simulink model "modelo_planta_CODESYS"  (R2025b)
settings: Solver=FixedStepAuto  StartTime=0.0  StopTime=inf  FixedStep=Ts2  MaxStep=1e-3  RelTol=1e-3
undefined symbols (not defined in the file): ah_max, at_max, bcx, bcy, bh_eq, bhb, bhEb, bhwu, bt, bt_eq, btb, btw, g, Hc, ih, it, Jh_eq, Jt_eq, Kcy, khwu, Ki_h, Ki_t, Kp_h, Kp_t, Kpos_h, Kpos_t, Ktw, lambda, Lh, Lh0, lh_0, Lt, magnitude, Mc_max, Ms, Mt, rhd, rtd, tau_hm, tau_tm, Thb_Max, ThEb_Max, Thm_0, Thm_Max, titahm_0, titatm_0, Ts0, Ts1, Ts2, Ttb_Max, Ttm_0, Ttm_Max, vh_0, vlx_0, vly_0, vt_0, vt_max, Wc, whm_0, whm_rated ... (+11)
libraries: simulink x10, opcualib x7, sl3dlib x1, simulink_extras x1, dspnetwork x1
(part 1 of 2)
settings Model: SimulationMode=accelerator  Creator=Nahuel  LastModifiedBy=nahue
settings SolverCC: ZeroCrossControl=DisableAll
settings DebuggingCC: UnderSpecifiedDimensionMsg=warning
settings SFSimCC: SimTargetLang=C++  SimDLTargetLibrary=mkl-dnn
settings RTWCC: GPUComputeCapability=3.5

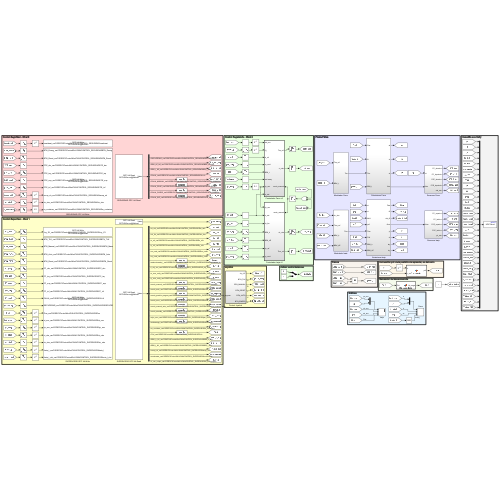
[thumbnail: Simulink's stored preview of the top-level diagram]
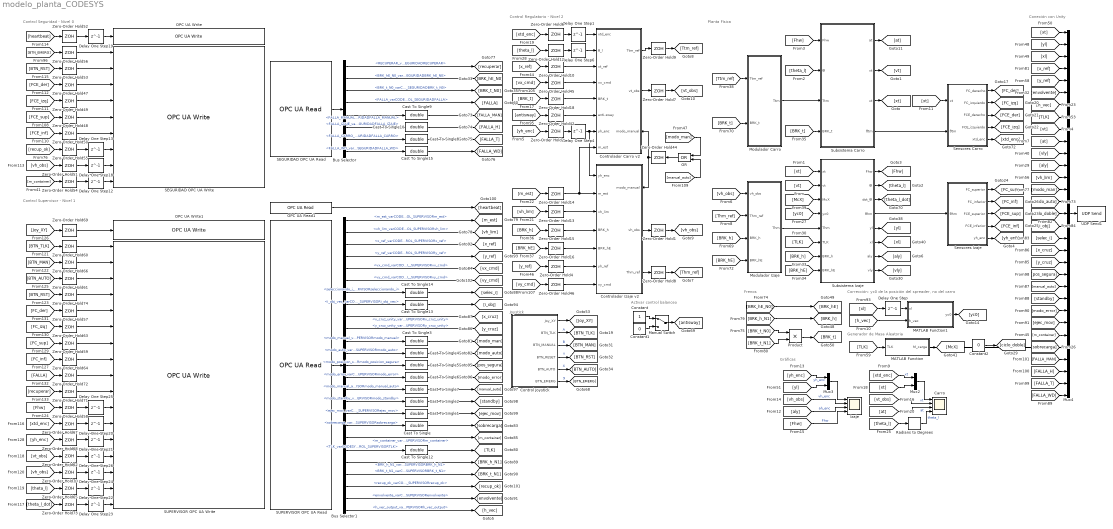
== system modelo_planta_CODESYS ==
  note: Activar control balanceo
  note: Generador de Masa Aleatoria
  note: Frenos
  note: Corrección: yc0 de la posición del spreader, no del carro
  note: Joystick
  note: Control Regulatorio - Nivel 2
  note: Conexión con Unity
  note: Planta Física
  note: Gráficas
  note: Control Seguridad - Nivel 0
  note: Control Supervisor - Nivel 1
  Bus Selector : BusSelector  OutputSignals=RECUPERAR_varCODESYSControlWinV3X64CONTROL_SEGURIDADRECUPERAR,BRK_hE_N0_varCODESYSControlWinV3X64CONTROL_SEGURIDADBRK_hE_N0,BRK_t_N0_varCODESYSControlWinV3X64CONTROL_SEGURIDADBRK_t_N0,FALLA_varCODESYSControlWinV3X64CONTROL_SEGURIDADFALLA,FALLA_MANUAL_varCODESYSControlWinV3X64CONTROL_SEGURIDADFALLA_MANUAL,FALLA_IZAJE_varCODESYSControlWinV3X64CONTROL_SEGURIDADFALLA_IZAJE,FALLA_CARRO_varCODESYSControlWinV3X64CONTROL_SEGURIDADFALLA_CARRO,FALLA_WD_varCODESYSControlWinV3X64CONTROL_SEGURIDADFALLA_WD
  Bus Selector1 : BusSelector  OutputSignals=m_est_varCODESYSControlWinV3X64CONTROL_SUPERVISORm_est,vh_lim_varCODESYSControlWinV3X64CONTROL_SUPERVISORvh_lim,x_ref_varCODESYSControlWinV3X64CONTROL_SUPERVISORx_ref,y_ref_varCODESYSControlWinV3X64CONTROL_SUPERVISORy_ref,vx_cmd_varCODESYSControlWinV3X64CONTROL_SUPERVISORvx_cmd,vy_cmd_varCODESYSControlWinV3X64CONTROL_SUPERVISORvy_cmd,seleccionando_i_varCODESYSControlWinV3X64CONTROL_SUPERVISORseleccionando_i,i_obj_vec_varCODESYSControlWinV3X64CONTROL_SUPERVISORi_obj_vec,x_cruz_unity_varCODESYSControlWinV3X64CONTROL_SUPERVISORx_cruz_unity,y_cruz_unity_varCODESYSControlWinV3X64CONTROL_SUPERVISORy_cruz_unity,modo_manual_varCODESYSControlWinV3X64CONTROL_SUPERVISORmodo_manual,modo_auto_varCODESYSControlWinV3X64CONTROL_SUPERVISORmodo_auto,modo_posicion_segura_varCODESYSControlWinV3X64CONTROL_SUPERVISORmodo_posicion_segura,modo_error_varCODESYSControlWinV3X64CONTROL_SUPERVISORmodo_error,modo_manual_auto_varCODESYSControlWinV3X64CONTROL_SUPERVISORmodo_manual_auto,modo_standby_varCODESYSControlWinV3X64CONTROL_SUPERVISORmodo_standby,ejec_mov_varCODESYSControlWinV3X64CONTROL_SUPERVISORejec_mov,sobrecarga_varCODESYSControlWinV3X64CONTROL_SUPERVISORsobrecarga,m_container_varCODESYSControlWinV3X64CONTROL_SUPERVISORm_container,TLK_varCODESYSControlWinV3X64CONTROL_SUPERVISORTLK,BRK_h_N1_varCODESYSControlWinV3X64CONTROL_SUPERVISORBRK_h_N1,BRK_t_N1_varCODESYSControlWinV3X64CONTROL_SUPERVISORBRK_t_N1,recup_ok_varCODESYSControlWinV3X64CONTROL_SUPERVISORrecup_ok,envolvente_varCODESYSControlWinV3X64CONTROL_SUPERVISORenvolvente,h_vec_output_varCODESYSControlWinV3X64CONTROL_SUPERVISORh_vec_output
  Carro : Scope  NumInputPorts=4
      settings: AxesScalingNumUpdates=5  ActiveDisplayYMinimum=-26.90845  ActiveDisplayYMaximum=42.17601
  Cast To Single{,1..10,12..15} (15 alike) : DataTypeConversion  OutDataTypeStr=double  SaturateOnIntegerOverflow=off  RndMeth=Floor
  Constant : Constant
  Constant1 : Constant  Value=0
  Constant2 : Constant  Value=0
  "Control Joystick " : Subsystem  TreatAsAtomicUnit=on  SystemSampleTime=Ts2
  Controlador Carro v2 : Subsystem  Priority=3  TreatAsAtomicUnit=on  SystemSampleTime=Ts2
      settings: PortSchema="{\"entries\":[{\"content\":{\"sides\":[{\"content\":{\"connectorIds\":[\"In1\",\"In2\",\"In3\",\"In4\",\"In5\",\"In6\",\"In7\",\"In8\"]},\"type\":\"ConnectorPlacement.EquallySpacedRectSide\",\"uuid\":\"cec1db83-79e7-401c-9c5a-62bfe309052c\"},{\"content\":{\"connectorIds\":[\"Out1\",\"Out2\",\"In9\"],\"side\":\"RIGHT\"},\"type\":\"ConnectorPlacement.EquallySpacedRectSide\",\"uuid\":\"570b393c-e744-4def-bec0-7a29fbc05550\"},{\"content\":{\"side\":\"TOP\"},\"type\":\"ConnectorPlacement.EquallySpacedRectSide\",\"uuid\":\"ce77deb8-7996-49cb-8f1a-144112ebd13f\"}]},\"type\":\"ConnectorPlacement.EquallySpacedConnector\",\"uuid\":\"f3fbcf0d-9250-48f2-9b40-44fd72963ab4\"}],\"packageUris\":[\"http://schema.mathworks.com/mf0/Connector/R2020b\"],\"version\":\"1.0\"}"
  Controlador Izaje v2 : Subsystem  Priority=3  TreatAsAtomicUnit=on  SystemSampleTime=Ts2
      settings: PortSchema="{\"entries\":[{\"content\":{\"sides\":[{\"content\":{\"connectorIds\":[\"In1\",\"In2\",\"In3\",\"In4\",\"In5\",\"In6\",\"In7\"]},\"type\":\"ConnectorPlacement.EquallySpacedRectSide\",\"uuid\":\"22fc4638-29ab-445f-b4f3-d8ad1dc2dec6\"},{\"content\":{\"connectorIds\":[\"In8\",\"Out1\",\"Out2\"],\"side\":\"RIGHT\"},\"type\":\"ConnectorPlacement.EquallySpacedRectSide\",\"uuid\":\"5bc2e66a-532f-4a2d-8b33-72ae52e90077\"},{\"content\":{\"side\":\"TOP\"},\"type\":\"ConnectorPlacement.EquallySpacedRectSide\",\"uuid\":\"2db62695-ea1c-4a55-b954-e8d85fe38ca0\"}]},\"type\":\"ConnectorPlacement.EquallySpacedConnector\",\"uuid\":\"0df15d49-0909-4287-a965-a213712e4789\"}],\"packageUris\":[\"http://schema.mathworks.com/mf0/Connector/R2020b\"],\"version\":\"1.0\"}"
  Delay One Step : Delay  DelayLength=1  InitialCondition=xl_0
  Delay One Step1 : Delay  DelayLength=1  InitialCondition=xtd_0
  Delay One Step{6,12..13,18..19,22..24,26} (9 alike) : Delay  DelayLength=1  InitialCondition=0
  Delay One Step20 : Delay  DelayLength=1  InitialCondition=xt_0
  Delay One Step21 : Delay  DelayLength=1  InitialCondition=yh_0
  Delay One Step25 : Delay  DelayLength=1
  Delay One Step4 : Delay  DelayLength=1  InitialCondition=yh_0
  Izaje : Scope  NumInputPorts=4
      settings: ActiveDisplayYMinimum=-22.31965  ActiveDisplayYMaximum=45.47272
  MATLAB Function : MATLAB Function  TreatAsAtomicUnit=on
  MATLAB Function1 : MATLAB Function  TreatAsAtomicUnit=on
  Manual Switch : ManualSwitch
  Modulador Carro : Subsystem
  Modulador Izaje : Subsystem
  Mux2 : Mux  Inputs=2
  Mux3 : Mux  Inputs=2
  Mux4 : Mux  Inputs=31
  OPC UA Read1 : opcualib/OPC UA Read  SelectedServer=OPCUAServer@Nahuel  ServerList=OPCUAServer@Nahuel  NodeList={ '1', 'heartbeat', '4', '|var|CODESYS Control Win V3 x64.CONTROL_SUPERVISOR.heartbeat', '0' }  ShowQualityPort=off  ShowTimestampPort=off  ShowTimestampPortAs=Seconds since start  SampleTime=Ts1
  OPC UA Write : opcualib/OPC UA Write  SelectedServer=OPCUAServer@Nahuel  ServerList=OPCUAServer@Nahuel  SampleTime=Ts0  NodeList={ '1', 'heartbeat', '4', '|var|CODESYS Control Win V3 x64.CONTROL_SEGURIDAD.heartbeat', '0' }
  OPC UA Write1 : opcualib/OPC UA Write  SelectedServer=OPCUAServer@Nahuel  ServerList=OPCUAServer@Nahuel  SampleTime=Ts1  NodeList={ '1', 'Joy_XY', '4', '|var|CODESYS Control Win V3 x64.CONTROL_SUPERVISOR.Joy_XY', '0' }
  OR : Logic  Operator=OR  IconShape=distinctive  AllPortsSameDT=off  OutDataTypeStr=boolean
  Product : Product
  Radians to Degrees : simulink_extras/Transformations/Radians to Degrees
  SEGURIDAD OPC UA Read : opcualib/OPC UA Read  SelectedServer=OPCUAServer@Nahuel  ServerList=OPCUAServer@Nahuel  NodeList={ '1', 'RECUPERAR', '4', '|var|CODESYS Control Win V3 x64.CONTROL_SEGURIDAD.RECUPERAR', '0'; '2', 'BRK_hE_N0', '4', '|var|CODESYS Control Win V3 x64.CONTROL_SEGURIDAD.BRK_hE_N0', '0'; '3', 'BRK_t_N0', '4', '|var|CODESYS Control Win V3 x64.CONTROL_SEGURIDAD.BRK_t_N0', '0'; '4', 'FALLA', '4', '|var|CODESYS Control Win V3 x64.CONTROL_SEGURIDAD.FALLA', '0'; '5', 'FALLA_MANUAL', '4', '|var|CODESYS Control Win V3 x64.CONTROL_SEGURIDAD.FALLA_MANUAL', '0'; '6', 'FALLA_IZAJE', '4', '|var|CODESYS Control Win V3 x64.CONTROL_SEGURIDAD.FALLA_IZAJE', '0'; '7', 'FALLA_CARRO', '4', '|var|CODESYS Control Win V3 x64.CONTROL_SEGURIDAD.FALLA_CARRO', '0'; '8', 'FALLA_WD', '4', '|var|CODESYS Control Win V3 x64.CONTROL_SEGURIDAD.FALLA_WD', '0' }  ShowQualityPort=off  ShowTimestampPort=off  ShowTimestampPortAs=Seconds since start  SampleTime=0.1
  SEGURIDAD OPC UA Write : opcualib/OPC UA Write  SelectedServer=OPCUAServer@Nahuel  ServerList=OPCUAServer@Nahuel  SampleTime=0.1  NodeList={ '1', 'BTN_Emerg', '4', '|var|CODESYS Control Win V3 x64.CONTROL_SEGURIDAD.BTN_Emerg', '0'; '2', 'BTN_Reset', '4', '|var|CODESYS Control Win V3 x64.CONTROL_SEGURIDAD.BTN_Reset', '0'; '3', 'FCE_der', '4', '|var|CODESYS Control Win V3 x64.CONTROL_SEGURIDAD.FCE_der', '0'; '4', 'FCE_izq', '4', '|var|CODESYS Control Win V3 x64.CONTROL_SEGURIDAD.FCE_izq', '0'; '5', 'FCE_sup', '4', '|var|CODESYS Control Win V3 x64.CONTROL_SEGURIDAD.FCE_sup', '0'; '6', 'FCE_inf', '4', '|var|CODESYS Control Win V3 x64.CONTROL_SEGURIDAD.FCE_inf', '0'; '7', 'recup_ok', '4', '|var|CODESYS Control Win V3 x64.CONTROL_SEGURIDAD.recup_ok', '0'; '8', 'vh_obs', '4', '|var|CODESYS Control Win V3 x64.CONTROL_SEGURIDAD.vh_obs', '0'; '9', 'm_container', '4', '|var|CODESYS Control Win V3 x64.CONTROL_SEGURIDAD.m_container', '0' }
  SUPERVISOR OPC UA Read : opcualib/OPC UA Read  SelectedServer=OPCUAServer@Nahuel  ServerList=OPCUAServer@Nahuel  NodeList={ '1', 'm_est', '4', '|var|CODESYS Control Win V3 x64.CONTROL_SUPERVISOR.m_est', '0'; '2', 'vh_lim', '4', '|var|CODESYS Control Win V3 x64.CONTROL_SUPERVISOR.vh_lim', '0'; '3', 'x_ref', '4', '|var|CODESYS Control Win V3 x64.CONTROL_SUPERVISOR.x_ref', '0'; '4', 'y_ref', '4', '|var|CODESYS Control Win V3 x64.CONTROL_SUPERVISOR.y_ref', '0'; '5', 'vx_cmd', '4', '|var|CODESYS Control Win V3 x64.CONTROL_SUPERVISOR.vx_cmd', '0'; '6', 'vy_cmd', '4', '|var|CODESYS Control Win V3 x64.CONTROL_SUPERVISOR.vy_cmd', '0'; '7', 'seleccionando_i', '4', '|var|CODESYS Control Win V3 x64.CONTROL_SUPERVISOR.seleccionando_i', '0'; '8', 'i_obj_vec', '4', '|var|CODESYS Control Win V3 x64.CONTROL_SUPERVISOR.i_obj_vec', '0'; '9', 'x_cruz_unity', '4', '|var|CODESYS Control Win V3 x64.CONTROL_SUPERVISOR.x_cruz_unity', '0'; '10', 'y_cruz_unity', '4', '|var|CODESYS Control Win V3 x64.CONTROL_SUPERVISOR.y_cruz_unity', '0'; '11', 'modo_manual', '4', '|var|CODESYS Control Win V3 x64.CONTROL_SUPERVISOR.modo_manual', '0'; '12', 'modo_auto', '4', '|var|CODESYS Control Win V3 x64.CONTROL_SUPERVISOR.modo_auto', '0'; '13', 'modo_posicion_segura', '4', '|var|CODESYS Control Win V3 x64.CONTROL_SUPERVISOR.modo_posicion_segura', '0'; '14', 'modo_error', '4', '|var|CODESYS Control Win V3 x64.CONTROL_SUPERVISOR.modo_error', '0'; '15', 'modo_manual_auto', '4', '|var|CODESYS Control Win V3 x64.CONTROL_SUPERVISOR.modo_manual_auto', '0'; '16', 'modo_standby', '4', '|var|CODESYS Control Win V3 x64.CONTROL_SUPERVISOR.modo_standby', '0'; '17', 'ejec_mov', '4', '|var|CODESYS Control Win V3 x64.CONTROL_SUPERVISOR.ejec_mov', '0'; '18', 'sobrecarga', '4', '|var|CODESYS Control Win V3 x64.CONTROL_SUPERVISOR.sobrecarga', '0'; '19', 'm_container', '4', '|var|CODESYS Control Win V3 x64.CONTROL_SUPERVISOR.m_container', '0'; '20', 'TLK', '4', '|var|CODESYS Control Win V3 x64.CONTROL_SUPERVISOR.TLK', '0'; '21', 'BRK_h_N1', '4', '|var|CODESYS Control Win V3 x64.CONTROL_SUPERVISOR.BRK_h_N1', '0'; '22', 'BRK_t_N1', '4', '|var|CODESYS Control Win V3 x64.CONTROL_SUPERVISOR.BRK_t_N1', '0'; '23', 'recup_ok', '4', '|var|CODESYS Control Win V3 x64.CONTROL_SUPERVISOR.recup_ok', '0'; '24', 'envolvente', '4', '|var|CODESYS Control Win V3 x64.CONTROL_SUPERVISOR.envolvente', '0'; '25', 'h_vec_output', '4', '|var|CODESYS Control Win V3 x64.CONTROL_SUPERVISOR.h_vec_output', '0' }  ShowQualityPort=off  ShowTimestampPort=off  ShowTimestampPortAs=Seconds since start  SampleTime=0.1
  SUPERVISOR OPC UA Write : opcualib/OPC UA Write  SelectedServer=OPCUAServer@Nahuel  ServerList=OPCUAServer@Nahuel  SampleTime=0.1  NodeList={ '1', 'BTN_TLK', '4', '|var|CODESYS Control Win V3 x64.CONTROL_SUPERVISOR.BTN_TLK', '0'; '2', 'BTN_Manual', '4', '|var|CODESYS Control Win V3 x64.CONTROL_SUPERVISOR.BTN_Manual', '0'; '3', 'BTN_Auto', '4', '|var|CODESYS Control Win V3 x64.CONTROL_SUPERVISOR.BTN_Auto', '0'; '4', 'BTN_Reset', '4', '|var|CODESYS Control Win V3 x64.CONTROL_SUPERVISOR.BTN_Reset', '0'; '5', 'FC_der', '4', '|var|CODESYS Control Win V3 x64.CONTROL_SUPERVISOR.FC_der', '0'; '6', 'FC_izq', '4', '|var|CODESYS Control Win V3 x64.CONTROL_SUPERVISOR.FC_izq', '0'; '7', 'FC_sup', '4', '|var|CODESYS Control Win V3 x64.CONTROL_SUPERVISOR.FC_sup', '0'; '8', 'FC_inf', '4', '|var|CODESYS Control Win V3 x64.CONTROL_SUPERVISOR.FC_inf', '0'; '9', 'FALLA', '4', '|var|CODESYS Control Win V3 x64.CONTROL_SUPERVISOR.FALLA', '0'; '10', 'RECUPERAR', '4', '|var|CODESYS Control Win V3 x64.CONTROL_SUPERVISOR.RECUPERAR', '0'; '11', 'Fhw', '4', '|var|CODESYS Control Win V3 x64.CONTROL_SUPERVISOR.Fhw', '0'; '12', 'xt_enc', '4', '|var|CODESYS Control Win V3 x64.CONTROL_SUPERVISOR.xt_enc', '0'; '13', 'yh_enc', '4', '|var|CODESYS Control Win V3 x64.CONTROL_SUPERVISOR.yh_enc', '0'; '14', 'vt_obs', '4', '|var|CODESYS Control Win V3 x64.CONTROL_SUPERVISOR.vt_obs', '0'; '15', 'vh_obs', '4', '|var|CODESYS Control Win V3 x64.CONTROL_SUPERVISOR.vh_obs', '0'; '16', 'theta_l', '4', '|var|CODESYS Control Win V3 x64.CONTROL_SUPERVISOR.theta_l', '0'; '17', 'theta_l_dot', '4', '|var|CODESYS Control Win V3 x64.CONTROL_SUPERVISOR.theta_l_dot', '0' }
  Sensores Carro : Subsystem
  Sensores Izaje : Subsystem
  Subsistema Carro : Subsystem
  Subsistema Izaje : Subsystem
  UDP Send1 : dspnetwork/UDP Send  remoteURL='127.0.0.1'  remotePort=1234  localURL='0.0.0.0'  localPortSource=Automatically determine  localPort=-1  sendBufferSize=8192  sampletime=-1  blockPlatform=HOST  separateLengthPort=0
  Zero-Order Hold{1..2,4,6..10,12..16,18,42,44..46} (18 alike) : ZeroOrderHold  SampleTime=Ts2
  Zero-Order Hold{47..56} (10 alike) : ZeroOrderHold  SampleTime=Ts0
  Zero-Order Hold{57..74} (18 alike) : ZeroOrderHold  SampleTime=Ts1
  wires:
  [Thm_ref] -> Modulador Izaje/2(Thm_ref)
  [vh_obs] -> Izaje/2  "vh_enc"
  Sensores Izaje/2(FC_inferior) -> [FC_inf]
  [x_ref] -> Zero-Order Hold10/1
  Zero-Order Hold4/1 -> Controlador Izaje v2/6(yh_ref)
  Delay One Step4/1 -> Controlador Izaje v2/1(yh_enc), Controlador Carro v2/7(yh_enc)
  Sensores Izaje/5(yh_enc) -> [yh_enc]
  [BRK_hE] -> Subsistema Izaje/8(BRK_hE)
  Subsistema Izaje/1(Fhw) -> [Fhw]
  Controlador Izaje v2/2(Thm_ref) -> Zero-Order Hold8/1
  [xt] -> Sensores Carro/1(xt)
  [BRK_h] -> Subsistema Izaje/7(BRK_h)
  Sensores Carro/2(FC_izquierdo) -> [FC_izq]
  [m_est] -> Zero-Order Hold14/1
  Zero-Order Hold2/1 -> Delay One Step4/1
  Zero-Order Hold6/1 -> Delay One Step1/1
  Subsistema Carro/1(at) -> [at]
  [theta_l] -> Subsistema Carro/2(θl)
  [vt] -> Subsistema Izaje/2(vt)
  [xt] -> Subsistema Izaje/1(xt)
  Delay One Step1/1 -> Controlador Carro v2/1(xtd_enc)
  [aly] -> Izaje/3  "ah_enc"
  Zero-Order Hold8/1 -> [Thm_ref]
  [vh_lim] -> Zero-Order Hold13/1
  Zero-Order Hold10/1 -> Controlador Carro v2/3(xt_ref)
  Subsistema Carro/3(xt) -> [xt]
  [Fhw] -> Subsistema Carro/1(Fhw)
  Sensores Carro/4(FCE_izquierdo) -> [FCE_izq]
  [yh_enc] -> Zero-Order Hold2/1
  [xtd_enc] -> Zero-Order Hold6/1
  Zero-Order Hold9/1 -> [Ttm_ref]
  Controlador Carro v2/1(Ttm_ref) -> Zero-Order Hold9/1
  [TLK] -> Subsistema Izaje/6(TLK)
  Subsistema Izaje/4(θhm) -> Sensores Izaje/1(θhm)
  Subsistema Carro/4(θtm) -> Sensores Carro/2(θtm)
  Sensores Izaje/4(FCE_inferior) -> [FCE_inf]
  Sensores Izaje/3(FCE_superior) -> [FCE_sup]
  Sensores Izaje/1(FC_superior) -> [FC_sup]
  Sensores Carro/3(FCE_derecho) -> [FCE_der]
  Subsistema Izaje/2(θl) -> [theta_l]
  [McX] -> Subsistema Izaje/3(McX)
  Subsistema Carro/2(vt) -> [vt]
  Sensores Carro/1(FC_derecho) -> [FC_der]
  [BRK_t] -> Subsistema Carro/4(BRK_t)
  [BRK_h] -> Zero-Order Hold15/1
  [BRK_hE] -> Zero-Order Hold16/1
  [Ttm_ref] -> Modulador Carro/1(Ttm_ref)
  [BRK_t] -> Zero-Order Hold18/1
  [yh_enc] -> Mux3/1  "yh_enc"
  [vh_obs] -> Modulador Izaje/1(vh_obs)
  Delay One Step6/1 -> Controlador Carro v2/2(θ_l)
  [theta_l] -> Zero-Order Hold12/1
  Zero-Order Hold12/1 -> Delay One Step6/1
  Modulador Izaje/1(Thm) -> Subsistema Izaje/5(Thm)
  Modulador Carro/1(Ttm) -> Subsistema Carro/3(Ttm)
  [y_ref] -> Zero-Order Hold4/1
  Mux3/1 -> Izaje/1
  Subsistema Izaje/5(yl) -> [yl]
  Subsistema Izaje/6(xl) -> [xl]
  [Fhw] -> Izaje/4  "Fhw"
  Subsistema Izaje/7(aly) -> [aly]
  [yl] -> Mux3/2
  Zero-Order Hold13/1 -> Controlador Izaje v2/3(vh_lim)
  Zero-Order Hold14/1 -> Controlador Carro v2/8(m_est), Controlador Izaje v2/2(m_est)
  Zero-Order Hold15/1 -> Controlador Izaje v2/4(BRK_h)
  Zero-Order Hold16/1 -> Controlador Izaje v2/5(BRK_hE)
  Zero-Order Hold18/1 -> Controlador Carro v2/5(BRK_t)
  [BRK_h] -> Modulador Izaje/3(BRK_h)
  [BRK_hE] -> Modulador Izaje/4(BRK_hE)
  [BRK_t] -> Modulador Carro/2(BRK_t)
  [BRK_t_N0] -> Product/1
  [BRK_t_N1] -> Product/2
  [BRK_h_N1] -> [BRK_h]
  [BRK_hE_N0] -> [BRK_hE]
  Product/1 -> [BRK_t]
  "Control Joystick "/2(BTN_TLK) -> [BTN_TLK]  "A"
  "Control Joystick "/1(Joy_XY) -> [Joy_XY]
  Subsistema Izaje/8(vly) -> [vly]
  "Control Joystick "/5(BTN_AUTO) -> [BTN_AUTO]  "X"
  "Control Joystick "/4(BTN_RESET) -> [BTN_RST]  "Y"
  "Control Joystick "/3(BTN_MANUAL) -> [BTN_MAN]  "B"
  [TLK] -> MATLAB Function/1(TLK)
  MATLAB Function/1(M_carga) -> [McX]
  [vh_lim] -> Mux4/13
  [at] -> Mux4/10
  [vt] -> Mux4/9
  [xt] -> Mux4/1
  [envolvente] -> Mux4/6
  [vly] -> Mux4/11
  [h_vec] -> Mux4/7
  [yl] -> Mux4/2
  [y_ref] -> Mux4/5
  [TLK] -> Mux4/8
  [xl] -> Mux4/3
  [x_ref] -> Mux4/4
  Mux4/1 -> UDP Send1/1
  [modo_man] -> Mux4/14
  [modo_auto] -> Mux4/15
  [ciclo_doble] -> Mux4/16
  [i_obj] -> Mux4/17
  [selec_i] -> Mux4/18
  [x_cruz] -> Mux4/19
  [y_cruz] -> Mux4/20
  [pos_segura] -> Mux4/21
  [manual_auto] -> Mux4/22
  [standby] -> Mux4/23
  [modo_error] -> Mux4/24
  [ejec_mov] -> Mux4/25
  [m_container] -> Mux4/26
  [sobrecarga] -> Mux4/27
  MATLAB Function1/1(yc0) -> [yc0]
  [xl] -> Delay One Step/1
  Delay One Step/1 -> MATLAB Function1/1(xl)
  [h_vec] -> MATLAB Function1/2(h_vec)
  [yc0] -> Subsistema Izaje/4(yc0)
  [aly] -> Mux4/12
  [FALLA_MAN] -> Mux4/28
  [FALLA_H] -> Mux4/29
  [FALLA_T] -> Mux4/30
  [FALLA_WD] -> Mux4/31
  "Control Joystick "/6(BTN_EMERG) -> [BTN_EMERG]  "9"
  Zero-Order Hold42/1 -> Controlador Carro v2/6(anti-sway)
  [antisway] -> Zero-Order Hold42/1
  Mux2/1 -> Carro/1
  [theta_l] -> Radians to Degrees/1
  [xt] -> Mux2/2
  [vt_obs] -> Carro/2  "vt"
  Radians to Degrees/1 -> Carro/4  "theta_l"
  [at] -> Carro/3  "at"
  [xtd_enc] -> Mux2/1  "xt"
  Subsistema Izaje/3(dot_θl) -> [theta_l_dot]
  Zero-Order Hold44/1 -> Controlador Carro v2/9(modo_manual), Controlador Izaje v2/8(modo_manual)
  [vx_cmd] -> Zero-Order Hold45/1
  Zero-Order Hold45/1 -> Controlador Carro v2/4(vx_cmd)
  [vy_cmd] -> Zero-Order Hold46/1
  Zero-Order Hold46/1 -> Controlador Izaje v2/7(vy_cmd)
  [modo_man] -> OR/1
  [manual_auto] -> OR/2
  OR/1 -> Zero-Order Hold44/1
  Controlador Carro v2/2(vt_obs) -> Zero-Order Hold7/1
  Zero-Order Hold7/1 -> [vt_obs]
  Sensores Carro/5(xtd_enc) -> [xtd_enc]
  Controlador Izaje v2/1(vh_obs) -> Zero-Order Hold1/1
  Zero-Order Hold1/1 -> [vh_obs]
  Constant/1 -> Manual Switch/1
  Manual Switch/1 -> [antisway]
  Constant1/1 -> Manual Switch/2
  Constant2/1 -> [ciclo_doble]
  SEGURIDAD OPC UA Read/1 -> Bus Selector/1
  Zero-Order Hold55/1 -> Delay One Step13/1
  [FCE_inf] -> Zero-Order Hold50/1
  [FCE_der] -> Zero-Order Hold47/1
  [m_container] -> Zero-Order Hold54/1
  Zero-Order Hold54/1 -> Delay One Step12/1
  [BTN_RST] -> Zero-Order Hold53/1
  [vh_obs] -> Zero-Order Hold51/1
  [FCE_izq] -> Zero-Order Hold49/1
  Zero-Order Hold51/1 -> Delay One Step18/1
  [recup_ok] -> Zero-Order Hold55/1
  [BTN_EMERG] -> Zero-Order Hold56/1
  [FCE_sup] -> Zero-Order Hold48/1
  Delay One Step12/1 -> SEGURIDAD OPC UA Write/9
  Delay One Step18/1 -> SEGURIDAD OPC UA Write/8
  Bus Selector/1 -> [recuperar]  "<RECUPERAR_varCODESYSControlWinV3X64CONTROL_SEGURIDADRECUPERAR>"
  Bus Selector/2 -> [BRK_hE_N0]  "<BRK_hE_N0_varCODESYSControlWinV3X64CONTROL_SEGURIDADBRK_hE_N0>"
  Bus Selector/3 -> [BRK_t_N0]  "<BRK_t_N0_varCODESYSControlWinV3X64CONTROL_SEGURIDADBRK_t_N0>"
  Bus Selector/4 -> [FALLA]  "<FALLA_varCODESYSControlWinV3X64CONTROL_SEGURIDADFALLA>"
  Bus Selector/5 -> Cast To Single9/1  "<FALLA_MANUAL_varCODESYSControlWinV3X64CONTROL_SEGURIDADFALLA_MANUAL>"
  Bus Selector/6 -> Cast To Single10/1  "<FALLA_IZAJE_varCODESYSControlWinV3X64CONTROL_SEGURIDADFALLA_IZAJE>"
  Bus Selector/7 -> Cast To Single8/1  "<FALLA_CARRO_varCODESYSControlWinV3X64CONTROL_SEGURIDADFALLA_CARRO>"
  Bus Selector/8 -> Cast To Single15/1  "<FALLA_WD_varCODESYSControlWinV3X64CONTROL_SEGURIDADFALLA_WD>"
  Zero-Order Hold56/1 -> SEGURIDAD OPC UA Write/1
  Zero-Order Hold53/1 -> SEGURIDAD OPC UA Write/2
  Zero-Order Hold47/1 -> SEGURIDAD OPC UA Write/3
  Zero-Order Hold49/1 -> SEGURIDAD OPC UA Write/4
  Zero-Order Hold48/1 -> SEGURIDAD OPC UA Write/5
  Zero-Order Hold50/1 -> SEGURIDAD OPC UA Write/6
  Delay One Step13/1 -> SEGURIDAD OPC UA Write/7
  Cast To Single8/1 -> [FALLA_T]
  Cast To Single10/1 -> [FALLA_H]
  Cast To Single9/1 -> [FALLA_MAN]
  [yh_enc] -> Zero-Order Hold68/1
  [vh_obs] -> Zero-Order Hold70/1
  [FC_izq] -> Zero-Order Hold63/1
  [theta_l_dot] -> Zero-Order Hold73/1
  Zero-Order Hold68/1 -> Delay One Step21/1
  [FALLA] -> Zero-Order Hold72/1
  [BTN_MAN] -> Zero-Order Hold66/1
  [FC_der] -> Zero-Order Hold57/1
  Zero-Order Hold73/1 -> Delay One Step23/1
  Zero-Order Hold65/1 -> Delay One Step22/1
  [FC_inf] -> Zero-Order Hold64/1
  [BTN_TLK] -> Zero-Order Hold60/1
  Zero-Order Hold62/1 -> Delay One Step26/1
  [Fhw] -> Zero-Order Hold58/1
  [BTN_AUTO] -> Zero-Order Hold61/1
  [theta_l] -> Zero-Order Hold65/1
  [xtd_enc] -> Zero-Order Hold67/1
  [BTN_RST] -> Zero-Order Hold74/1
  [FC_sup] -> Zero-Order Hold59/1
  Zero-Order Hold70/1 -> Delay One Step24/1
  Zero-Order Hold58/1 -> Delay One Step25/1
  Zero-Order Hold67/1 -> Delay One Step20/1
  [recuperar] -> Zero-Order Hold71/1
  [vt_obs] -> Zero-Order Hold62/1
  Zero-Order Hold66/1 -> SUPERVISOR OPC UA Write/2
  Zero-Order Hold61/1 -> SUPERVISOR OPC UA Write/3
  Zero-Order Hold74/1 -> SUPERVISOR OPC UA Write/4
  Zero-Order Hold57/1 -> SUPERVISOR OPC UA Write/5
  Zero-Order Hold63/1 -> SUPERVISOR OPC UA Write/6
  Zero-Order Hold59/1 -> SUPERVISOR OPC UA Write/7
  Zero-Order Hold64/1 -> SUPERVISOR OPC UA Write/8
  Zero-Order Hold72/1 -> SUPERVISOR OPC UA Write/9
  Zero-Order Hold71/1 -> SUPERVISOR OPC UA Write/10
  Zero-Order Hold60/1 -> SUPERVISOR OPC UA Write/1
  Delay One Step25/1 -> SUPERVISOR OPC UA Write/11
  Delay One Step20/1 -> SUPERVISOR OPC UA Write/12
  Delay One Step21/1 -> SUPERVISOR OPC UA Write/13
  Delay One Step26/1 -> SUPERVISOR OPC UA Write/14
  Delay One Step24/1 -> SUPERVISOR OPC UA Write/15
  Delay One Step22/1 -> SUPERVISOR OPC UA Write/16
  Delay One Step23/1 -> SUPERVISOR OPC UA Write/17
  Bus Selector1/1 -> [m_est]  "<m_est_varCODESYSControlWinV3X64CONTROL_SUPERVISORm_est>"
  Bus Selector1/2 -> [vh_lim]  "<vh_lim_varCODESYSControlWinV3X64CONTROL_SUPERVISORvh_lim>"
  Bus Selector1/3 -> [x_ref]  "<x_ref_varCODESYSControlWinV3X64CONTROL_SUPERVISORx_ref>"
  Bus Selector1/4 -> [y_ref]  "<y_ref_varCODESYSControlWinV3X64CONTROL_SUPERVISORy_ref>"
  Bus Selector1/5 -> [vx_cmd]  "<vx_cmd_varCODESYSControlWinV3X64CONTROL_SUPERVISORvx_cmd>"
  Bus Selector1/6 -> [vy_cmd]  "<vy_cmd_varCODESYSControlWinV3X64CONTROL_SUPERVISORvy_cmd>"
  Bus Selector1/7 -> Cast To Single14/1  "<seleccionando_i_varCODESYSControlWinV3X64CONTROL_SUPERVISORseleccionando_i>"
  Bus Selector1/8 -> Cast To Single13/1  "<i_obj_vec_varCODESYSControlWinV3X64CONTROL_SUPERVISORi_obj_vec>"
  Bus Selector1/9 -> [x_cruz]  "<x_cruz_unity_varCODESYSControlWinV3X64CONTROL_SUPERVISORx_cruz_unity>"
  Bus Selector1/10 -> [y_cruz]  "<y_cruz_unity_varCODESYSControlWinV3X64CONTROL_SUPERVISORy_cruz_unity>"
  Bus Selector1/11 -> Cast To Single3/1  "<modo_manual_varCODESYSControlWinV3X64CONTROL_SUPERVISORmodo_manual>"
  Bus Selector1/12 -> Cast To Single4/1  "<modo_auto_varCODESYSControlWinV3X64CONTROL_SUPERVISORmodo_auto>"
  Bus Selector1/13 -> Cast To Single5/1  "<modo_posicion_segura_varCODESYSControlWinV3X64CONTROL_SUPERVISORmodo_posicion_segura>"
  Bus Selector1/14 -> Cast To Single6/1  "<modo_error_varCODESYSControlWinV3X64CONTROL_SUPERVISORmodo_error>"
  Bus Selector1/15 -> Cast To Single7/1  "<modo_manual_auto_varCODESYSControlWinV3X64CONTROL_SUPERVISORmodo_manual_auto>"
  Bus Selector1/16 -> Cast To Single2/1  "<modo_standby_varCODESYSControlWinV3X64CONTROL_SUPERVISORmodo_standby>"
  Bus Selector1/17 -> Cast To Single1/1  "<ejec_mov_varCODESYSControlWinV3X64CONTROL_SUPERVISORejec_mov>"
  Bus Selector1/18 -> Cast To Single/1  "<sobrecarga_varCODESYSControlWinV3X64CONTROL_SUPERVISORsobrecarga>"
  Bus Selector1/19 -> [m_container]  "<m_container_varCODESYSControlWinV3X64CONTROL_SUPERVISORm_container>"
  Bus Selector1/20 -> Cast To Single12/1  "<TLK_varCODESYSControlWinV3X64CONTROL_SUPERVISORTLK>"
  Bus Selector1/21 -> [BRK_h_N1]  "<BRK_h_N1_varCODESYSControlWinV3X64CONTROL_SUPERVISORBRK_h_N1>"
  Bus Selector1/22 -> [BRK_t_N1]  "<BRK_t_N1_varCODESYSControlWinV3X64CONTROL_SUPERVISORBRK_t_N1>"
  Bus Selector1/23 -> [recup_ok]  "<recup_ok_varCODESYSControlWinV3X64CONTROL_SUPERVISORrecup_ok>"
  Bus Selector1/24 -> [envolvente]  "<envolvente_varCODESYSControlWinV3X64CONTROL_SUPERVISORenvolvente>"
  Bus Selector1/25 -> [h_vec]  "<h_vec_output_varCODESYSControlWinV3X64CONTROL_SUPERVISORh_vec_output>"
  SUPERVISOR OPC UA Read/1 -> Bus Selector1/1
  Cast To Single3/1 -> [modo_man]
  Cast To Single4/1 -> [modo_auto]
  Cast To Single5/1 -> [pos_segura]
  Cast To Single6/1 -> [modo_error]
  Cast To Single7/1 -> [manual_auto]
  Cast To Single2/1 -> [standby]
  Cast To Single1/1 -> [ejec_mov]
  Cast To Single/1 -> [sobrecarga]
  Cast To Single15/1 -> [FALLA_WD]
  Cast To Single12/1 -> [TLK]
  Cast To Single13/1 -> [i_obj]
  Cast To Single14/1 -> [selec_i]
  OPC UA Read1/1 -> [heartbeat]
  [heartbeat] -> Zero-Order Hold52/1
  Zero-Order Hold52/1 -> Delay One Step19/1
  Delay One Step19/1 -> OPC UA Write/1
  [Joy_XY] -> Zero-Order Hold69/1
  Zero-Order Hold69/1 -> OPC UA Write1/1

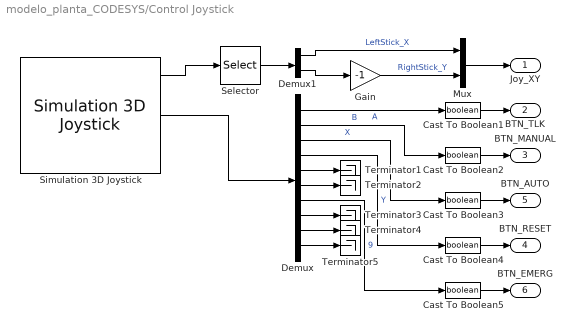
== system modelo_planta_CODESYS/Control Joystick  ==
  Cast To Boolean{1..5} (5 alike) : DataTypeConversion  OutDataTypeStr=boolean  SaturateOnIntegerOverflow=off  RndMeth=Floor
  Demux : Demux  Outputs=10
  Demux1 : Demux  Outputs=2
  Gain : Gain  Gain=-1
  Mux : Mux  Inputs=2
  Selector : Selector  InputPortWidth=5  IndexOptions=Index vector (dialog)  Indices=[1 5]  OutputSizes=1
  Simulation 3D Joystick : sl3dlib/Simulation 3D/Hardware Interface/Simulation 3D Joystick  joyid=1  adjustports=on  forcefeed=off
  Terminator{1..5} (5 alike) : Terminator
  Joy_XY : Outport
  BTN_TLK : Outport  Port=2
  BTN_MANUAL : Outport  Port=3
  BTN_RESET : Outport  Port=4
  BTN_AUTO : Outport  Port=5
  BTN_EMERG : Outport  Port=6
  wires:
  Demux/1 -> Cast To Boolean1/1  "A"
  Demux1/2 -> Gain/1
  Demux1/1 -> Mux/1  "LeftStick_X"
  Selector/1 -> Demux1/1
  Simulation 3D Joystick/1 -> Selector/1
  Gain/1 -> Mux/2  "RightStick_Y"
  Simulation 3D Joystick/2 -> Demux/1
  Demux/2 -> Cast To Boolean2/1  "B"
  Demux/3 -> Cast To Boolean3/1  "X"
  Demux/4 -> Cast To Boolean4/1  "Y"
  Mux/1 -> Joy_XY/1
  Demux/5 -> Terminator1/1
  Demux/6 -> Terminator2/1
  Demux/8 -> Terminator3/1
  Demux/9 -> Terminator4/1
  Demux/10 -> Terminator5/1
  Demux/7 -> Cast To Boolean5/1  "9"
  Cast To Boolean1/1 -> BTN_TLK/1
  Cast To Boolean2/1 -> BTN_MANUAL/1
  Cast To Boolean3/1 -> BTN_AUTO/1
  Cast To Boolean4/1 -> BTN_RESET/1
  Cast To Boolean5/1 -> BTN_EMERG/1

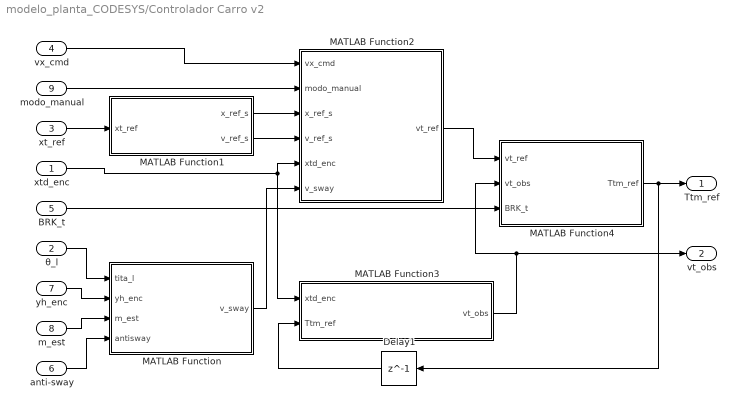
== system modelo_planta_CODESYS/Controlador Carro v2 ==
  xtd_enc : Inport
  θ_l : Inport  Port=2
  xt_ref : Inport  Port=3
  vx_cmd : Inport  Port=4
  BRK_t : Inport  Port=5
  anti-sway : Inport  Port=6
  yh_enc : Inport  Port=7
  m_est : Inport  Port=8
  modo_manual : Inport  Port=9
  Delay1 : Delay  DelayLength=1  InitialCondition=Ttm_0
  MATLAB Function : MATLAB Function  TreatAsAtomicUnit=on
  MATLAB Function1 : MATLAB Function  TreatAsAtomicUnit=on
  MATLAB Function2 : MATLAB Function  TreatAsAtomicUnit=on
  MATLAB Function3 : MATLAB Function  TreatAsAtomicUnit=on
  MATLAB Function4 : MATLAB Function  TreatAsAtomicUnit=on
  Ttm_ref : Outport
  vt_obs : Outport  Port=2
  wires:
  xt_ref/1 -> MATLAB Function1/1(xt_ref)
  BRK_t/1 -> MATLAB Function4/3(BRK_t)
  yh_enc/1 -> MATLAB Function/2(yh_enc)
  θ_l/1 -> MATLAB Function/1(tita_l)
  anti-sway/1 -> MATLAB Function/4(antisway)
  vx_cmd/1 -> MATLAB Function2/1(vx_cmd)
  modo_manual/1 -> MATLAB Function2/2(modo_manual)
  xtd_enc/1 -> MATLAB Function3/1(xtd_enc), MATLAB Function2/5(xtd_enc)
  m_est/1 -> MATLAB Function/3(m_est)
  MATLAB Function1/1(x_ref_s) -> MATLAB Function2/3(x_ref_s)
  MATLAB Function1/2(v_ref_s) -> MATLAB Function2/4(v_ref_s)
  MATLAB Function/1(v_sway) -> MATLAB Function2/6(v_sway)
  MATLAB Function2/1(vt_ref) -> MATLAB Function4/1(vt_ref)
  MATLAB Function3/1(vt_obs) -> vt_obs/1, MATLAB Function4/2(vt_obs)
  MATLAB Function4/1(Ttm_ref) -> Ttm_ref/1, Delay1/1
  Delay1/1 -> MATLAB Function3/2(Ttm_ref)

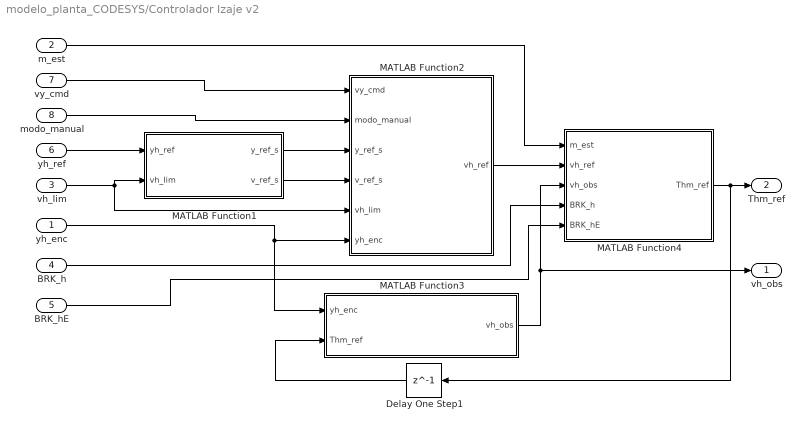
== system modelo_planta_CODESYS/Controlador Izaje v2 ==
  yh_enc : Inport
  m_est : Inport  Port=2
  vh_lim : Inport  Port=3
  BRK_h : Inport  Port=4
  BRK_hE : Inport  Port=5
  yh_ref : Inport  Port=6
  vy_cmd : Inport  Port=7
  modo_manual : Inport  Port=8
  Delay One Step1 : Delay  DelayLength=1  InitialCondition=Thm_0
  MATLAB Function1 : MATLAB Function  TreatAsAtomicUnit=on
  MATLAB Function2 : MATLAB Function  TreatAsAtomicUnit=on
  MATLAB Function3 : MATLAB Function  TreatAsAtomicUnit=on
  MATLAB Function4 : MATLAB Function  TreatAsAtomicUnit=on
  vh_obs : Outport
  Thm_ref : Outport  Port=2
  wires:
  yh_ref/1 -> MATLAB Function1/1(yh_ref)
  vh_lim/1 -> MATLAB Function2/5(vh_lim), MATLAB Function1/2(vh_lim)
  MATLAB Function1/1(y_ref_s) -> MATLAB Function2/3(y_ref_s)
  MATLAB Function1/2(v_ref_s) -> MATLAB Function2/4(v_ref_s)
  vy_cmd/1 -> MATLAB Function2/1(vy_cmd)
  modo_manual/1 -> MATLAB Function2/2(modo_manual)
  yh_enc/1 -> MATLAB Function3/1(yh_enc), MATLAB Function2/6(yh_enc)
  m_est/1 -> MATLAB Function4/1(m_est)
  MATLAB Function2/1(vh_ref) -> MATLAB Function4/2(vh_ref)
  MATLAB Function3/1(vh_obs) -> MATLAB Function4/3(vh_obs), vh_obs/1
  BRK_h/1 -> MATLAB Function4/4(BRK_h)
  BRK_hE/1 -> MATLAB Function4/5(BRK_hE)
  MATLAB Function4/1(Thm_ref) -> Delay One Step1/1, Thm_ref/1
  Delay One Step1/1 -> MATLAB Function3/2(Thm_ref)

== system modelo_planta_CODESYS/Modulador Carro ==
  Ttm_ref : Inport
  BRK_t : Inport  Port=2
  Constant : Constant  Value=Ttm_Max
  Gain1 : Gain  Gain=-1
  Gain2 : Gain  Gain=1/tau_tm
  Integrator : Integrator  InitialCondition=Ttm_0
  Product : Product
  Saturation Dynamic : simulink/Discontinuities/Saturation Dynamic  OutMin=[]  OutMax=[]  OutDataTypeStr=Inherit: Same as second input  OutDataType=fixdt(1, 16)  OutScaling=2^-10  DoSatur=off
  Sum : Sum  Inputs=|+-
  Ttm : Outport
  wires:
  Constant/1 -> Saturation Dynamic/1, Gain1/1
  Gain1/1 -> Saturation Dynamic/3
  Saturation Dynamic/1 -> Sum/1  "Ttm_lim"
  Sum/1 -> Gain2/1
  Gain2/1 -> Integrator/1
  Integrator/1 -> Ttm/1, Sum/2
  Ttm_ref/1 -> Product/1
  BRK_t/1 -> Product/2
  Product/1 -> Saturation Dynamic/2

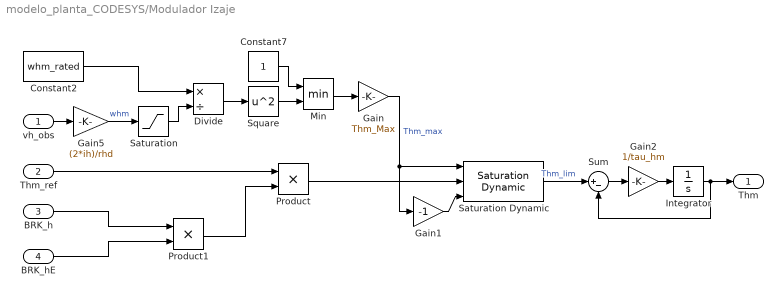
== system modelo_planta_CODESYS/Modulador Izaje ==
  vh_obs : Inport
  Thm_ref : Inport  Port=2
  BRK_h : Inport  Port=3
  BRK_hE : Inport  Port=4
  Constant2 : Constant  Value=whm_rated
  Constant7 : Constant
  Divide : Product  Inputs=*/
  Gain : Gain  Gain=Thm_Max
  Gain1 : Gain  Gain=-1
  Gain2 : Gain  Gain=1/tau_hm
  Gain5 : Gain  Gain=(2*ih)/rhd
  Integrator : Integrator  InitialCondition=Thm_0
  Min : MinMax  Inputs=2
  Product : Product
  Product1 : Product
  Saturation : Saturate  UpperLimit=inf  LowerLimit=whm_rated
  Saturation Dynamic : simulink/Discontinuities/Saturation Dynamic  OutMin=[]  OutMax=[]  OutDataTypeStr=Inherit: Same as second input  OutDataType=fixdt(1, 16)  OutScaling=2^-10  DoSatur=off
  Square : Math  Operator=square
  Sum : Sum  Inputs=|+-
  Thm : Outport
  wires:
  Constant2/1 -> Divide/1
  Min/1 -> Gain/1
  Constant7/1 -> Min/1
  Gain/1 -> Gain1/1, Saturation Dynamic/1  "Thm_max"
  Saturation/1 -> Divide/2
  Square/1 -> Min/2
  Divide/1 -> Square/1
  vh_obs/1 -> Gain5/1
  Gain1/1 -> Saturation Dynamic/3
  Saturation Dynamic/1 -> Sum/1  "Thm_lim"
  Sum/1 -> Gain2/1
  Gain2/1 -> Integrator/1
  Integrator/1 -> Thm/1, Sum/2
  Thm_ref/1 -> Product/1
  BRK_h/1 -> Product1/1
  Product/1 -> Saturation Dynamic/2
  BRK_hE/1 -> Product1/2
  Product1/1 -> Product/2
  Gain5/1 -> Saturation/1  "whm"

== system modelo_planta_CODESYS/Sensores Carro ==
  xt : Inport
  θtm : Inport  Port=2
  Encoder Carro : Subsystem
  Fines de carrera carro (rieles) : Subsystem
  FC_derecho : Outport
  FC_izquierdo : Outport  Port=2
  FCE_derecho : Outport  Port=3
  FCE_izquierdo : Outport  Port=4
  xtd_enc : Outport  Port=5
  wires:
  Fines de carrera carro (rieles)/1(FC_derecho) -> FC_derecho/1
  θtm/1 -> Encoder Carro/1(θtm)
  Fines de carrera carro (rieles)/2(FC_izquierdo) -> FC_izquierdo/1
  Fines de carrera carro (rieles)/3(FCE_derecho) -> FCE_derecho/1
  Fines de carrera carro (rieles)/4(FCE_izquierdo) -> FCE_izquierdo/1
  xt/1 -> Fines de carrera carro (rieles)/1(xt)
  Encoder Carro/1(xtd_enc) -> xtd_enc/1

== system modelo_planta_CODESYS/Sensores Izaje ==
  θhm : Inport
  Encoder Izaje : Subsystem
  Fines de carrera izaje (tambor) : Subsystem
  FC_superior : Outport
  FC_inferior : Outport  Port=2
  FCE_superior : Outport  Port=3
  FCE_inferior : Outport  Port=4
  yh_enc : Outport  Port=5
  wires:
  Fines de carrera izaje (tambor)/1(FC_superior) -> FC_superior/1
  Fines de carrera izaje (tambor)/4(FCE_inferior) -> FCE_inferior/1
  Fines de carrera izaje (tambor)/2(FC_inferior) -> FC_inferior/1
  Encoder Izaje/1(yh_enc) -> Fines de carrera izaje (tambor)/1(y_enc), yh_enc/1
  θhm/1 -> Encoder Izaje/1(θhm)
  Fines de carrera izaje (tambor)/3(FCE_superior) -> FCE_superior/1

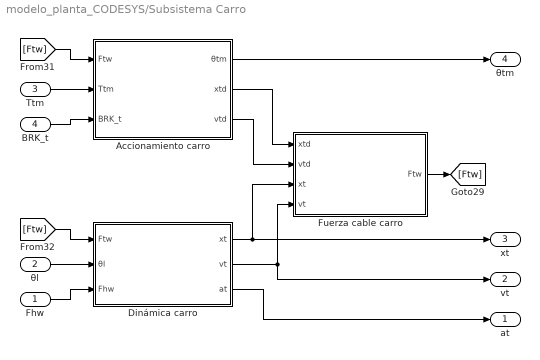
== system modelo_planta_CODESYS/Subsistema Carro ==
  Fhw : Inport
  θl : Inport  Port=2
  Ttm : Inport  Port=3
  BRK_t : Inport  Port=4
  Accionamiento carro : Subsystem
  Dinámica carro : Subsystem
  Fuerza cable carro : Subsystem
  at : Outport
  vt : Outport  Port=2
  xt : Outport  Port=3
  θtm : Outport  Port=4
  wires:
  [Ftw] -> Accionamiento carro/1(Ftw)
  Accionamiento carro/1(θtm) -> θtm/1
  Dinámica carro/1(xt) -> Fuerza cable carro/3(xt), xt/1
  BRK_t/1 -> Accionamiento carro/3(BRK_t)
  [Ftw] -> Dinámica carro/1(Ftw)
  θl/1 -> Dinámica carro/2(θl)
  Ttm/1 -> Accionamiento carro/2(Ttm)
  Fuerza cable carro/1(Ftw) -> [Ftw]
  Dinámica carro/2(vt) -> Fuerza cable carro/4(vt), vt/1
  Accionamiento carro/2(xtd) -> Fuerza cable carro/1(xtd)
  Accionamiento carro/3(vtd) -> Fuerza cable carro/2(vtd)
  Fhw/1 -> Dinámica carro/3(Fhw)
  Dinámica carro/3(at) -> at/1

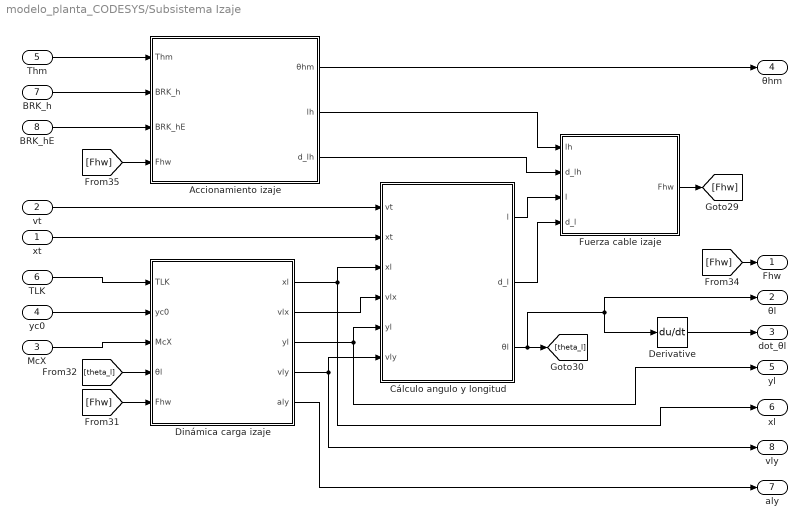
== system modelo_planta_CODESYS/Subsistema Izaje ==
  xt : Inport
  vt : Inport  Port=2
  McX : Inport  Port=3
  yc0 : Inport  Port=4
  Thm : Inport  Port=5
  TLK : Inport  Port=6
  BRK_h : Inport  Port=7
  BRK_hE : Inport  Port=8
  Accionamiento izaje : Subsystem
  Cálculo angulo y longitud : Subsystem
  Derivative : Derivative
  Dinámica carga izaje : Subsystem
  Fuerza cable izaje : Subsystem
  Fhw : Outport
  θl : Outport  Port=2
  dot_θl : Outport  Port=3
  θhm : Outport  Port=4
  yl : Outport  Port=5
  xl : Outport  Port=6
  aly : Outport  Port=7
  vly : Outport  Port=8
  wires:
  vt/1 -> Cálculo angulo y longitud/1(vt)
  Accionamiento izaje/2(lh) -> Fuerza cable izaje/1(lh)
  yc0/1 -> Dinámica carga izaje/2(yc0)
  McX/1 -> Dinámica carga izaje/3(McX)
  Dinámica carga izaje/4(vly) -> vly/1, Cálculo angulo y longitud/6(vly)
  [Fhw] -> Accionamiento izaje/4(Fhw)
  [theta_l] -> Dinámica carga izaje/4(θl)
  xt/1 -> Cálculo angulo y longitud/2(xt)
  BRK_h/1 -> Accionamiento izaje/2(BRK_h)
  Dinámica carga izaje/1(xl) -> Cálculo angulo y longitud/3(xl), xl/1
  Dinámica carga izaje/2(vlx) -> Cálculo angulo y longitud/4(vlx)
  Fuerza cable izaje/1(Fhw) -> [Fhw]
  Cálculo angulo y longitud/1(l) -> Fuerza cable izaje/3(l)
  Accionamiento izaje/1(θhm) -> θhm/1
  Cálculo angulo y longitud/3(θl) -> θl/1, Derivative/1, [theta_l]
  TLK/1 -> Dinámica carga izaje/1(TLK)
  [Fhw] -> Dinámica carga izaje/5(Fhw)
  BRK_hE/1 -> Accionamiento izaje/3(BRK_hE)
  Thm/1 -> Accionamiento izaje/1(Thm)
  Dinámica carga izaje/3(yl) -> Cálculo angulo y longitud/5(yl), yl/1
  Cálculo angulo y longitud/2(d_l) -> Fuerza cable izaje/4(d_l)
  Accionamiento izaje/3(d_lh) -> Fuerza cable izaje/2(d_lh)
  Dinámica carga izaje/5(aly) -> aly/1
  [Fhw] -> Fhw/1
  Derivative/1 -> dot_θl/1

== system modelo_planta_CODESYS/Sensores Carro/Encoder Carro ==
  θtm : Inport
  Gain1 : Gain  Gain=rtd/it
  xtd_enc : Outport
  wires:
  θtm/1 -> Gain1/1
  Gain1/1 -> xtd_enc/1

== system modelo_planta_CODESYS/Sensores Carro/Fines de carrera carro (rieles) ==
  xt : Inport
  Compare To Constant : simulink/Logic and Bit Operations/Compare To Constant  relop=>=  const=xt_max  OutDataTypeStr=boolean
  Compare To Constant1 : simulink/Logic and Bit Operations/Compare To Constant  relop=>=  const=xt_max+0.5  OutDataTypeStr=boolean
  Compare To Constant2 : simulink/Logic and Bit Operations/Compare To Constant  relop=<=  const=xt_min  OutDataTypeStr=boolean
  Compare To Constant3 : simulink/Logic and Bit Operations/Compare To Constant  relop=<=  const=xt_min-0.5  OutDataTypeStr=boolean
  FC_derecho : Outport
  FC_izquierdo : Outport  Port=2
  FCE_derecho : Outport  Port=3
  FCE_izquierdo : Outport  Port=4
  wires:
  Compare To Constant2/1 -> FC_izquierdo/1
  xt/1 -> Compare To Constant/1, Compare To Constant1/1, Compare To Constant2/1, Compare To Constant3/1
  Compare To Constant3/1 -> FCE_izquierdo/1
  Compare To Constant1/1 -> FCE_derecho/1
  Compare To Constant/1 -> FC_derecho/1

== system modelo_planta_CODESYS/Sensores Izaje/Encoder Izaje ==
  θhm : Inport
  Gain3 : Gain  Gain=rhd/(2*ih)
  yh_enc : Outport
  wires:
  θhm/1 -> Gain3/1
  Gain3/1 -> yh_enc/1

== system modelo_planta_CODESYS/Sensores Izaje/Fines de carrera izaje (tambor) ==
  y_enc : Inport
  Compare To Constant4 : simulink/Logic and Bit Operations/Compare To Constant  relop=>=  const=yh_max  OutDataTypeStr=boolean
  Compare To Constant5 : simulink/Logic and Bit Operations/Compare To Constant  relop=>=  const=yh_max+0.5  OutDataTypeStr=boolean
  Compare To Constant6 : simulink/Logic and Bit Operations/Compare To Constant  relop=<=  const=yh_min  OutDataTypeStr=boolean
  Compare To Constant7 : simulink/Logic and Bit Operations/Compare To Constant  relop=<=  const=yh_min-0.5  OutDataTypeStr=boolean
  FC_superior : Outport
  FC_inferior : Outport  Port=2
  FCE_superior : Outport  Port=3
  FCE_inferior : Outport  Port=4
  wires:
  Compare To Constant7/1 -> FCE_inferior/1
  y_enc/1 -> Compare To Constant7/1, Compare To Constant6/1, Compare To Constant4/1, Compare To Constant5/1
  Compare To Constant6/1 -> FC_inferior/1
  Compare To Constant5/1 -> FCE_superior/1
  Compare To Constant4/1 -> FC_superior/1

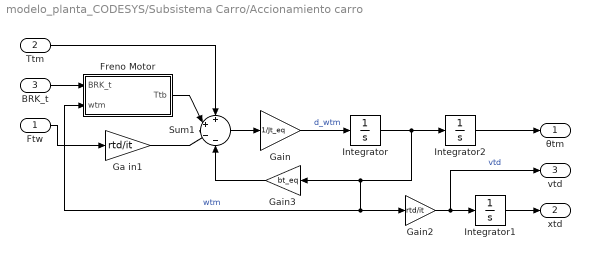
== system modelo_planta_CODESYS/Subsistema Carro/Accionamiento carro ==
  Ftw : Inport
  Ttm : Inport  Port=2
  BRK_t : Inport  Port=3
  Freno Motor : Subsystem
  Ga in1 : Gain  Gain=rtd/it
  Gain : Gain  Gain=1/Jt_eq
  Gain2 : Gain  Gain=rtd/it
  Gain3 : Gain  Gain=bt_eq
  Integrator : Integrator  InitialCondition=wtm_0
  Integrator1 : Integrator  InitialCondition=xtd_0
  Integrator2 : Integrator  InitialCondition=titatm_0
  Sum1 : Sum  Inputs=++--
  θtm : Outport
  xtd : Outport  Port=2
  vtd : Outport  Port=3
  wires:
  Sum1/1 -> Gain/1
  Integrator/1 -> Gain2/1, Freno Motor/2(wtm), Gain3/1, Integrator2/1  "wtm"
  Gain2/1 -> Integrator1/1, vtd/1  "vtd"
  Ttm/1 -> Sum1/1
  Gain/1 -> Integrator/1  "d_wtm"
  BRK_t/1 -> Freno Motor/1(BRK_t)
  Integrator1/1 -> xtd/1
  Ftw/1 -> Ga in1/1
  Ga in1/1 -> Sum1/3
  Freno Motor/1(Ttb) -> Sum1/2
  Gain3/1 -> Sum1/4
  Integrator2/1 -> θtm/1

== system modelo_planta_CODESYS/Subsistema Carro/Dinámica carro ==
  Ftw : Inport
  θl : Inport  Port=2
  Fhw : Inport  Port=3
  Gain : Gain  Gain=2
  Gain1 : Gain  Gain=1/Mt
  Gain2 : Gain  Gain=bt
  Integrator : Integrator  InitialCondition=vt_0
  Integrator1 : Integrator  InitialCondition=xt_0
  Product : Product
  Sin : Trigonometry
  Sum : Sum  Inputs=++-
  xt : Outport
  vt : Outport  Port=2
  at : Outport  Port=3
  wires:
  Gain1/1 -> at/1, Integrator/1  "dot_vt"
  Integrator/1 -> Gain2/1, vt/1, Integrator1/1  "vt"
  Gain2/1 -> Sum/3
  Sum/1 -> Gain1/1
  Integrator1/1 -> xt/1  "xt"
  Fhw/1 -> Gain/1
  Gain/1 -> Product/2
  θl/1 -> Sin/1
  Sin/1 -> Product/1
  Product/1 -> Sum/2  "F_coupling"
  Ftw/1 -> Sum/1

== system modelo_planta_CODESYS/Subsistema Carro/Fuerza cable carro ==
  xtd : Inport
  vtd : Inport  Port=2
  xt : Inport  Port=3
  vt : Inport  Port=4
  Gain : Gain  Gain=Ktw
  Gain1 : Gain  Gain=btw
  Sum : Sum  Inputs=+-
  Sum1 : Sum
  Sum2 : Sum  Inputs=+-
  Ftw : Outport
  wires:
  xtd/1 -> Sum/1
  Gain1/1 -> Sum1/2
  Sum/1 -> Gain/1
  xt/1 -> Sum/2
  Sum2/1 -> Gain1/1
  Gain/1 -> Sum1/1
  vt/1 -> Sum2/2
  Sum1/1 -> Ftw/1  "Ftw"
  vtd/1 -> Sum2/1

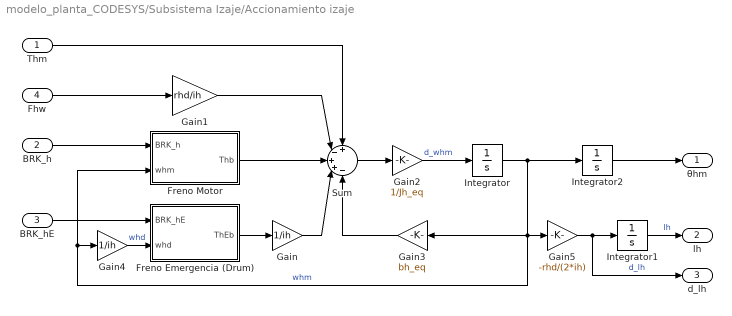
== system modelo_planta_CODESYS/Subsistema Izaje/Accionamiento izaje ==
  Thm : Inport
  BRK_h : Inport  Port=2
  BRK_hE : Inport  Port=3
  Fhw : Inport  Port=4
  Freno Emergencia (Drum) : Subsystem
  Freno Motor : Subsystem
  Gain : Gain  Gain=1/ih
  Gain1 : Gain  Gain=rhd/ih
  Gain2 : Gain  Gain=1/Jh_eq
  Gain3 : Gain  Gain=bh_eq
  Gain4 : Gain  Gain=1/ih
  Gain5 : Gain  Gain=-rhd/(2*ih)
  Integrator : Integrator  InitialCondition=whm_0
  Integrator1 : Integrator  InitialCondition=lh_0
  Integrator2 : Integrator  InitialCondition=titahm_0
  Sum : Sum  Inputs=+-++-
  θhm : Outport
  lh : Outport  Port=2
  d_lh : Outport  Port=3
  wires:
  Gain5/1 -> d_lh/1, Integrator1/1  "d_lh"
  Integrator/1 -> Gain3/1, Freno Motor/2(whm), Gain4/1, Gain5/1, Integrator2/1  "whm"
  Freno Emergencia (Drum)/1(ThEb) -> Gain/1
  Gain3/1 -> Sum/5
  BRK_h/1 -> Freno Motor/1(BRK_h)
  Gain/1 -> Sum/4
  Gain2/1 -> Integrator/1  "d_whm"
  Sum/1 -> Gain2/1
  Gain4/1 -> Freno Emergencia (Drum)/2(whd)  "whd"
  BRK_hE/1 -> Freno Emergencia (Drum)/1(BRK_hE)
  Fhw/1 -> Gain1/1
  Freno Motor/1(Thb) -> Sum/3
  Gain1/1 -> Sum/2
  Integrator1/1 -> lh/1  "lh"
  Integrator2/1 -> θhm/1
  Thm/1 -> Sum/1

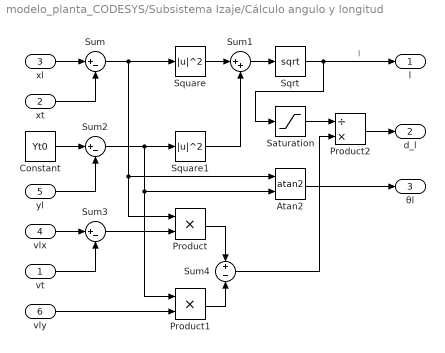
== system modelo_planta_CODESYS/Subsistema Izaje/Cálculo angulo y longitud ==
  vt : Inport
  xt : Inport  Port=2
  xl : Inport  Port=3
  vlx : Inport  Port=4
  yl : Inport  Port=5
  vly : Inport  Port=6
  Atan2 : Trigonometry  Operator=atan2
  Constant : Constant  Value=Yt0
  Product : Product
  Product1 : Product
  Product2 : Product  Inputs=/*
  Saturation : Saturate  UpperLimit=inf  LowerLimit=0.1
  Sqrt : Sqrt
  Square : Math  Operator=magnitude^2
  Square1 : Math  Operator=magnitude^2
  Sum : Sum  Inputs=|+-
  Sum1 : Sum  Inputs=|++
  Sum2 : Sum  Inputs=|+-
  Sum3 : Sum  Inputs=|+-
  Sum4 : Sum  Inputs=+-
  l : Outport
  d_l : Outport  Port=2
  θl : Outport  Port=3
  wires:
  Product2/1 -> d_l/1
  Sqrt/1 -> l/1, Saturation/1  "l"
  Sum1/1 -> Sqrt/1
  Sum2/1 -> Product1/1, Atan2/2, Square1/1
  Sum/1 -> Product/1, Atan2/1, Square/1
  yl/1 -> Sum2/2
  Atan2/1 -> θl/1
  vly/1 -> Product1/2
  xl/1 -> Sum/1
  Constant/1 -> Sum2/1
  Sum3/1 -> Product/2
  Square1/1 -> Sum1/2
  vt/1 -> Sum3/2
  Sum4/1 -> Product2/2
  vlx/1 -> Sum3/1
  xt/1 -> Sum/2
  Square/1 -> Sum1/1
  Product1/1 -> Sum4/2
  Product/1 -> Sum4/1
  Saturation/1 -> Product2/1

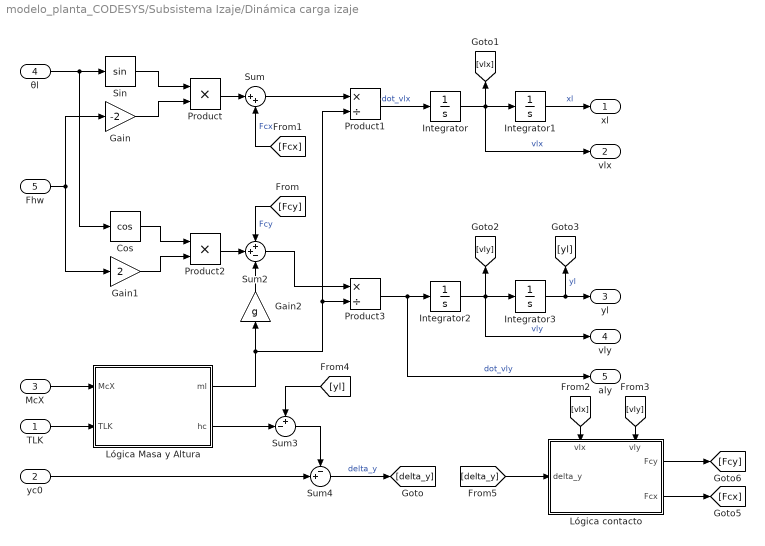
== system modelo_planta_CODESYS/Subsistema Izaje/Dinámica carga izaje ==
  TLK : Inport
  yc0 : Inport  Port=2
  McX : Inport  Port=3
  θl : Inport  Port=4
  Fhw : Inport  Port=5
  Cos : Trigonometry  Operator=cos
  Gain : Gain  Gain=-2
  Gain1 : Gain  Gain=2
  Gain2 : Gain  Gain=g
  Integrator : Integrator  InitialCondition=vlx_0
  Integrator1 : Integrator  InitialCondition=xl_0
  Integrator2 : Integrator  InitialCondition=vly_0
  Integrator3 : Integrator  InitialCondition=yl_0
  Lógica Masa y Altura : Subsystem
  Lógica contacto : Subsystem
      settings: PortSchema="{\"entries\":[{\"content\":{\"sides\":[{\"content\":{\"connectorIds\":[\"In1\"]},\"type\":\"ConnectorPlacement.EquallySpacedRectSide\",\"uuid\":\"20a8b2c4-d5cf-44ce-93ec-929b996a0905\"},{\"content\":{\"connectorIds\":[\"Out1\",\"Out2\"],\"side\":\"RIGHT\"},\"type\":\"ConnectorPlacement.EquallySpacedRectSide\",\"uuid\":\"396e1f2e-cf71-48dc-8d57-a3e2695dfff1\"},{\"content\":{\"connectorIds\":[\"In2\",\"In3\"],\"side\":\"TOP\"},\"type\":\"ConnectorPlacement.EquallySpacedRectSide\",\"uuid\":\"e66c0478-9682-41e1-9b77-d2d789a9c323\"}]},\"type\":\"ConnectorPlacement.EquallySpacedConnector\",\"uuid\":\"193dabd2-f524-433a-b6ef-c1cab585578e\"}],\"packageUris\":[\"http://schema.mathworks.com/mf0/Connector/R2020b\"],\"version\":\"1.0\"}"
  Product : Product
  Product1 : Product  Inputs=*/
  Product2 : Product
  Product3 : Product  Inputs=*/
  Sin : Trigonometry
  Sum : Sum  Inputs=|++
  Sum2 : Sum  Inputs=++-
  Sum3 : Sum  Inputs=+-|
  Sum4 : Sum  Inputs=-+|
  xl : Outport
  vlx : Outport  Port=2
  yl : Outport  Port=3
  vly : Outport  Port=4
  aly : Outport  Port=5
  wires:
  θl/1 -> Sin/1, Cos/1
  Integrator/1 -> vlx/1, Integrator1/1, [vlx]  "vlx"
  Sum3/1 -> Sum4/1
  Sin/1 -> Product/1
  Gain/1 -> Product/2
  [Fcy] -> Sum2/1  "Fcy"
  Integrator2/1 -> vly/1, Integrator3/1, [vly]  "vly"
  Integrator3/1 -> yl/1, [yl]  "yl"
  Fhw/1 -> Gain1/1, Gain/1
  [Fcx] -> Sum/2  "Fcx"
  Product/1 -> Sum/1
  Product1/1 -> Integrator/1  "dot_vlx"
  Gain2/1 -> Sum2/3
  Cos/1 -> Product2/1
  Gain1/1 -> Product2/2
  [yl] -> Sum3/1
  Product2/1 -> Sum2/2
  yc0/1 -> Sum4/2
  Sum2/1 -> Product3/1
  Product3/1 -> aly/1, Integrator2/1  "dot_vly"
  Sum/1 -> Product1/1
  Integrator1/1 -> xl/1  "xl"
  Sum4/1 -> [delta_y]  "delta_y"
  Lógica contacto/1(Fcy) -> [Fcy]
  Lógica contacto/2(Fcx) -> [Fcx]
  Lógica Masa y Altura/1(ml) -> Product1/2, Product3/2, Gain2/1
  McX/1 -> Lógica Masa y Altura/1(McX)
  TLK/1 -> Lógica Masa y Altura/2(TLK)
  Lógica Masa y Altura/2(hc) -> Sum3/2
  [vlx] -> Lógica contacto/2(vlx)
  [vly] -> Lógica contacto/3(vly)
  [delta_y] -> Lógica contacto/1(delta_y)

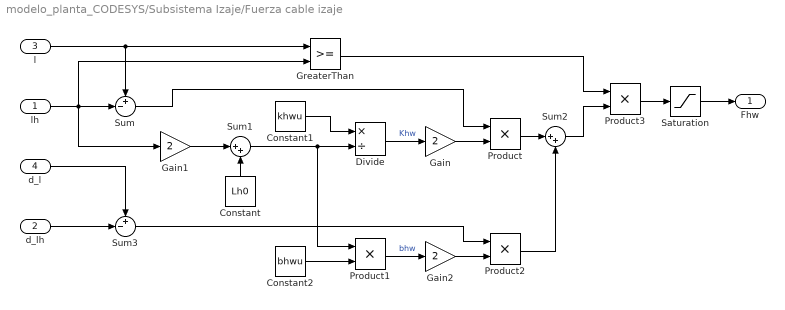
== system modelo_planta_CODESYS/Subsistema Izaje/Fuerza cable izaje ==
  lh : Inport
  d_lh : Inport  Port=2
  l : Inport  Port=3
  d_l : Inport  Port=4
  Constant : Constant  Value=Lh0
  Constant1 : Constant  Value=khwu
  Constant2 : Constant  Value=bhwu
  Divide : Product  Inputs=*/  RndMeth=Zero  SaturateOnIntegerOverflow=on
  Gain : Gain  Gain=2
  Gain1 : Gain  Gain=2
  Gain2 : Gain  Gain=2
  GreaterThan : RelationalOperator  OutDataTypeStr=boolean  RndMeth=Simplest  InputSameDT=off
  Product{,1..3} (4 alike) : Product
  Saturation : Saturate  UpperLimit=inf  LowerLimit=0
  Sum : Sum  Inputs=+-|
  Sum1 : Sum  Inputs=|++
  Sum2 : Sum  Inputs=|++
  Sum3 : Sum  Inputs=+-|
  Fhw : Outport
  wires:
  Constant/1 -> Sum1/2
  Constant2/1 -> Product1/2
  Sum1/1 -> Divide/2, Product1/1
  lh/1 -> Sum/2, GreaterThan/2, Gain1/1
  Product/1 -> Sum2/1
  Gain1/1 -> Sum1/1
  l/1 -> Sum/1, GreaterThan/1
  Product2/1 -> Sum2/2
  Product3/1 -> Saturation/1
  GreaterThan/1 -> Product3/1
  d_lh/1 -> Sum3/2
  Constant1/1 -> Divide/1
  Product1/1 -> Gain2/1  "bhw"
  Sum/1 -> Product/1
  Gain2/1 -> Product2/2
  Divide/1 -> Gain/1  "Khw"
  Sum2/1 -> Product3/2
  Sum3/1 -> Product2/1
  d_l/1 -> Sum3/1
  Gain/1 -> Product/2
  Saturation/1 -> Fhw/1

== system modelo_planta_CODESYS/Subsistema Carro/Accionamiento carro/Freno Motor ==
  BRK_t : Inport
  wtm : Inport  Port=2
  Constant : Constant  Value=0
  Gain3 : Gain  Gain=-Ttb_Max
  Gain4 : Gain  Gain=btb
  Switch : Switch  Criteria=u2 > Threshold  SaturateOnIntegerOverflow=off  InputSameDT=off
  Tanh : Trigonometry  Operator=tanh
  Ttb : Outport
  wires:
  BRK_t/1 -> Switch/2
  Constant/1 -> Switch/1
  wtm/1 -> Gain4/1
  Gain4/1 -> Tanh/1
  Tanh/1 -> Gain3/1
  Gain3/1 -> Switch/3
  Switch/1 -> Ttb/1

== system modelo_planta_CODESYS/Subsistema Izaje/Accionamiento izaje/Freno Emergencia (Drum) ==
  BRK_hE : Inport
  whd : Inport  Port=2
  Constant : Constant  Value=0
  Gain3 : Gain  Gain=-ThEb_Max
  Gain4 : Gain  Gain=bhEb
  Switch : Switch  Criteria=u2 > Threshold  SaturateOnIntegerOverflow=off  InputSameDT=off
  Tanh : Trigonometry  Operator=tanh
  ThEb : Outport
  wires:
  BRK_hE/1 -> Switch/2
  Gain3/1 -> Switch/3
  Constant/1 -> Switch/1
  whd/1 -> Gain4/1
  Gain4/1 -> Tanh/1
  Tanh/1 -> Gain3/1
  Switch/1 -> ThEb/1

== system modelo_planta_CODESYS/Subsistema Izaje/Accionamiento izaje/Freno Motor ==
  BRK_h : Inport
  whm : Inport  Port=2
  Constant : Constant  Value=0
  Gain3 : Gain  Gain=-Thb_Max
  Gain4 : Gain  Gain=bhb
  Switch : Switch  Criteria=u2 > Threshold  SaturateOnIntegerOverflow=off  InputSameDT=off
  Tanh : Trigonometry  Operator=tanh
  Thb : Outport
  wires:
  BRK_h/1 -> Switch/2
  Gain3/1 -> Switch/3
  Constant/1 -> Switch/1
  whm/1 -> Gain4/1
  Gain4/1 -> Tanh/1
  Tanh/1 -> Gain3/1
  Switch/1 -> Thb/1
